simulink model "Test_Model"  (R2020a)
settings: Solver=ode15s  StartTime=0.0  StopTime=15  RelTol=1e-3
libraries: simulink x2
settings Model: Creator=Matthew  LastModifiedBy=Matthew

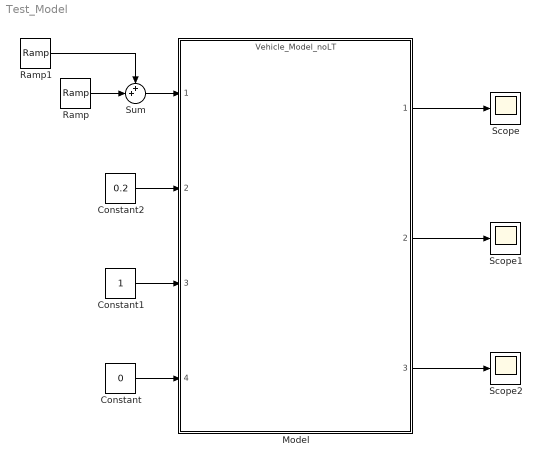
== system Test_Model ==
  Constant : Constant  Value=0  OutDataTypeStr=int8
  Constant1 : Constant
  Constant2 : Constant  Value=0.2
  Model : ModelReference  ModelNameDialog=Vehicle_Model_noLT  SimulationMode=Normal  ModelReferenceVersion=1.13
  Ramp : simulink/Sources/Ramp  slope=-0.5  start=2  InitialOutput=0
  Ramp1 : simulink/Sources/Ramp  slope=0.5  start=0  InitialOutput=0
  Scope : Scope
  Scope1 : Scope
  Scope2 : Scope
  Sum : Sum  Inputs=++|
  wires:
  Constant/1 -> Model/4
  Constant1/1 -> Model/3
  Constant2/1 -> Model/2
  Sum/1 -> Model/1
  Ramp/1 -> Sum/2
  Ramp1/1 -> Sum/1
  Model/1 -> Scope/1
  Model/2 -> Scope1/1
  Model/3 -> Scope2/1
